simulink model "sampleModel226"  (R2021b)
settings: Solver=VariableStepAuto  StartTime=0.0  StopTime=10.0  RelTol=1e-3
undefined symbols (not defined in the file or in its folder): DiscIntNeverNeededParam, Newton, Raphson
libraries: simulink x16, slpidlib x3
settings Model: Creator=user  LastModifiedBy=user

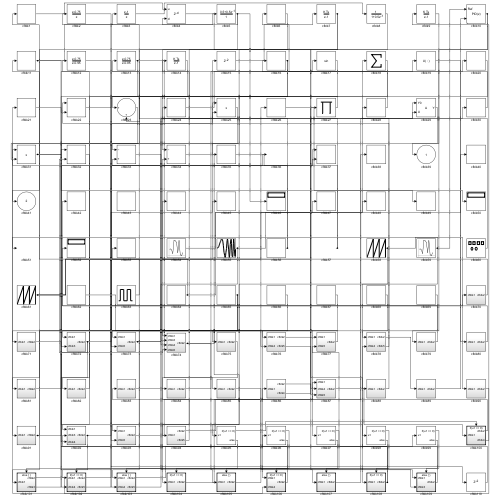
[thumbnail: Simulink's stored preview of the top-level diagram]
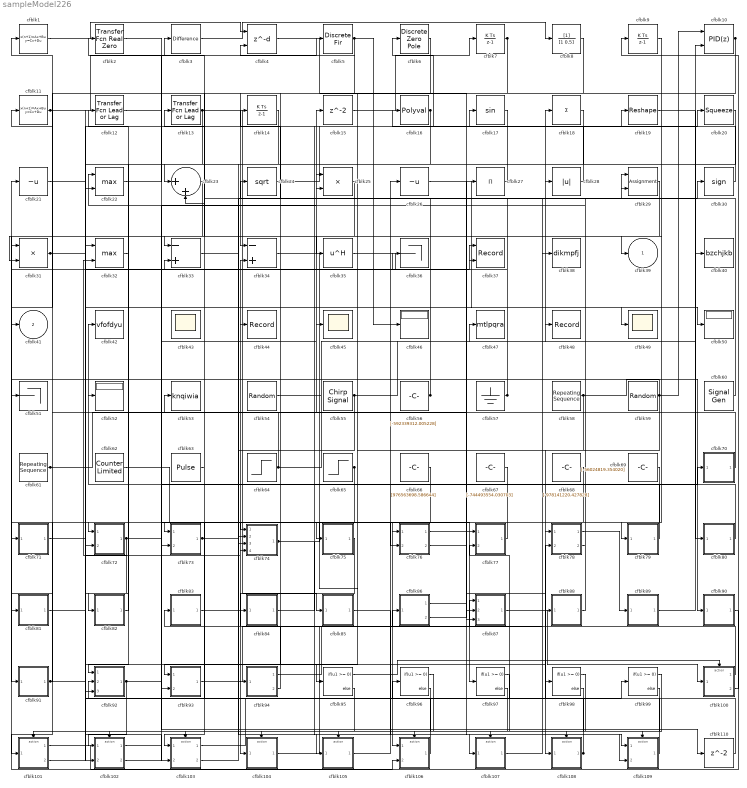
== system sampleModel226 ==
  cfblk1 : DiscreteStateSpace
  cfblk10 : slpidlib/PID Controller (2DOF)  Controller=PID  Form=Parallel  TimeDomain=Discrete-time  UseExternalTs=off  SampleTime=1  IntegratorMethod=Forward Euler  FilterMethod=Forward Euler  ControllerParametersSource=internal  P=1  I=1  D=0  UseFilter=on  N=100  b=1  c=1  TunerSelectOption=Transfer Function Based (PID Tuner App)  InitialConditionSource=internal  InitialConditionForIntegrator=0  InitialConditionForFilter=0  DifferentiatorICPrevScaledInput=0  ExternalReset=none  TrackingMode=off  Kt=1  LimitOutput=off  SatLimitsSource=internal  UpperSaturationLimit=inf  LowerSaturationLimit=-inf  LinearizeAsGain=off  AntiWindupMode=none  Kb=1  POutMin=[]  POutMax=[]  IOutMin=[]  IOutMax=[]  DOutMin=[]  DOutMax=[]  NOutMin=[]  NOutMax=[]  bOutMin=[]  bOutMax=[]  cOutMin=[]  cOutMax=[]  SumOutMin=[]  SumOutMax=[]  SaturationOutMin=[]  SaturationOutMax=[]  PParamMin=[]  PParamMax=[]  IParamMin=[]  IParamMax=[]  DParamMin=[]  DParamMax=[]  NParamMin=[]  NParamMax=[]  bParamMin=[]  bParamMax=[]  cParamMin=[]  cParamMax=[]  KbParamMin=[]  KbParamMax=[]  KtParamMin=[]  KtParamMax=[]  KbOutMin=[]  KbOutMax=[]  KtOutMin=[]  KtOutMax=[]  IntegratorOutMin=[]  IntegratorOutMax=[]  FilterOutMin=[]  FilterOutMax=[]  SumI1OutMin=[]  SumI1OutMax=[]  SumI2OutMin=[]  SumI2OutMax=[]  SumI3OutMin=[]  SumI3OutMax=[]  SumI4OutMin=[]  SumI4OutMax=[]  SumDOutMin=[]  SumDOutMax=[]  Sum1OutMin=[]  Sum1OutMax=[]  Sum2OutMin=[]  Sum2OutMax=[]  Sum3OutMin=[]  Sum3OutMax=[]  DifferentiatorOutMin=[]  DifferentiatorOutMax=[]  FilterDiffOutCoefMin=[]  FilterDiffOutCoefMax=[]  ReciprocalOutMin=[]  ReciprocalOutMax=[]  SumDenOutMin=[]  SumDenOutMax=[]  SumNumOutMin=[]  SumNumOutMax=[]  DivideOutMin=[]  DivideOutMax=[]  UdiffTsProdOutMin=[]  UdiffTsProdOutMax=[]  NTsProdOutMin=[]  NTsProdOutMax=[]  UintegralTsProdOutMin=[]  UintegralTsProdOutMax=[]  UngainTsProdOutMin=[]  UngainTsProdOutMax=[]  IntegratorContinuousStateAttributes=''  IntegratorStateMustResolveToSignalObject=off  IntegratorRTWStateStorageClass=Auto  FilterContinuousStateAttributes=''  FilterStateMustResolveToSignalObject=off  FilterRTWStateStorageClass=Auto  ParallelPVariant=InternalParameters  IdealPVariant=Disabled  IVariant=InternalParameters  DVariant=InternalParameters  bVariant=InternalParameters  cVariant=InternalParameters  IntegratorVariant=Discrete  SatVariant=Disabled  AWVariant=Passthrough  PCopyVariant=Disabled  TRVariant=Disabled  FdbkBlocksVariant=Forward  IdealPFdbkVariant=Disabled  SatFdbkVariant=Disabled  DerivativeFilterVariant=ForwardEulerFilter  NVariant=InternalParameters  NCopyVariant=Disabled  FilterICVariant=InternalICsFilter  IntegratorICVariant=InternalICs  ExternalResetVariant=Disabled  TRSumVariant=Passthrough  SumFdbkVariant=Disabled  SumVariant=Sum_PID  TsampFilterVariant=InternalTs  TsampNgainVariant=Passthrough  TsampIntegralVariant=Passthrough  ExternalSaturationOutDataTypeStr=Inherit: Same as second input
      settings: SourceProductBaseCode=SL
  cfblk100 : Subsystem  TreatAsAtomicUnit=on
  cfblk101 : Subsystem  TreatAsAtomicUnit=on
  cfblk102 : Subsystem  TreatAsAtomicUnit=on
  cfblk103 : Subsystem  TreatAsAtomicUnit=on
  cfblk104 : Subsystem  TreatAsAtomicUnit=on
  cfblk105 : Subsystem  TreatAsAtomicUnit=on
  cfblk106 : Subsystem  TreatAsAtomicUnit=on
  cfblk107 : Subsystem  TreatAsAtomicUnit=on
  cfblk108 : Subsystem  TreatAsAtomicUnit=on
  cfblk109 : Subsystem  TreatAsAtomicUnit=on
  cfblk11 : DiscreteStateSpace
  cfblk110 : Delay  SampleTime=1
  cfblk12 : simulink/Discrete/Transfer Fcn Lead or Lag  PoleZ=0.95  ZeroZ=0.75  ICPrevOutput=0.0  ICPrevInput=0.0  DoSatur=off
      settings: SourceProductBaseCode=SL
  cfblk13 : simulink/Discrete/Transfer Fcn Lead or Lag  PoleZ=0.95  ZeroZ=0.75  ICPrevOutput=0.0  ICPrevInput=0.0  DoSatur=off
      settings: SourceProductBaseCode=SL
  cfblk14 : DiscreteIntegrator  ICPrevOutput=DiscIntNeverNeededParam  ICPrevScaledInput=DiscIntNeverNeededParam
  cfblk15 : Delay  SampleTime=1
  cfblk16 : Polyval  Coefs=[ +2.081618890e-019, -1.441693666e-014, +4.719686976e-010, -8.536869453e-006, +1.621573104e-001, -8.087801117e+001 ]
  cfblk17 : Trigonometry
  cfblk18 : Sum  Inputs=+
  cfblk19 : Reshape
  cfblk2 : simulink/Discrete/Transfer Fcn Real Zero  ZeroZ=0.75  ICPrevInput=0.0  DoSatur=off
      settings: SourceProductBaseCode=SL
  cfblk20 : Squeeze
  cfblk21 : UnaryMinus
  cfblk22 : MinMax  Function=max  Inputs=2
  cfblk23 : Sum  Inputs=|++
  cfblk24 : Sqrt  SaturateOnIntegerOverflow=on
  cfblk25 : Product
  cfblk26 : UnaryMinus
  cfblk27 : Product  Inputs=*
  cfblk28 : Abs
  cfblk29 : Assignment  DiagnosticForDimensions=Warning  IndexOptions=Index vector (dialog)  Indices=1  OutputSizes=1
  cfblk3 : simulink/Discrete/Difference  ICPrevInput=0.0  OutMin=[]  OutMax=[]  OutDataTypeStr=Inherit: Inherit via back propagation  OutDataType=fixdt(1, 16)  OutScaling=2^-10  DoSatur=off
  cfblk30 : Signum
  cfblk31 : Product  Inputs=**
  cfblk32 : MinMax  Function=max  Inputs=2
  cfblk33 : Sum  Inputs=-+
  cfblk34 : Sum  Inputs=-+
  cfblk35 : Math  Operator=hermitian  SaturateOnIntegerOverflow=on
  cfblk36 : Terminator
  cfblk37 : Record  FileSettingsInternal="{\"entries\":[{\"content\":{\"excelSettings\":{\"content\":{},\"type\":\"Streamout.ExcelSettings\"}},\"type\":\"Streamout.FileSettingStorage\",\"uuid\":\"d36e2a6a-7d58-4cca-bbfa-2d4460a6e9a2\"}],\"packageUris\":[\"http://schema.mathworks.com/mf0/streamout_blocks/R2020a\"],\"version\":\"1.0\"}"  Layout=[1 1]  SignalsInternal="{\"entries\":[{\"content\":{\"signals\":[{\"content\":{\"blockPath\":[\"sampleModel226/cfblk37\"],\"channel\":[],\"dimensions\":[1],\"domain\":\"sampleModel226/cfblk37\",\"lineColor\":\"#a2142f\",\"plots\":[1],\"port\":1,\"sid\":[\"\"],\"signalID\":8845,\"signalName\":\"cfblk81\"},\"type\":\"RecordBlkView.Signal\",\"uuid\":\"4bfdb0e3-98e3-43bb-8b1d-080535746a11\"},{\"content\":{\"blockPath\":[\"sampleModel226/cfblk37\"],\"channel\":[],\"dimensions\":[1,1],\"domain\":\"sampleModel226/cfblk37\",\"lineColor\":\"#139fff\",\"plots\":[1],\"port\":2,\"sid\":[\"\"],\"signalID\":8849,\"signalName\":\"cfblk35\"},\"type\":\"RecordBlkView.Signal\",\"uuid\":\"6c2a1cae-b381-4225-acec-e32f350de892\"}]},\"type\":\"RecordBlkView.InputSignals\",\"uuid\":\"7360f588-8737-44e8-b6c5-5c4f20366708\"}],\"packageUris\":[\"http://schema.mathworks.com/mf0/streamout_blocks/R2020a\"],\"version\":\"1.0\"}"  VisualizationBindings="{\"xyplotplugin\":{\"info\":[{\"series\":[{\"bindingParametersList\":[{\"parameter\":\"X-Axis\",\"signalID\":8845,\"signalName\":\"cfblk81\"},{\"parameter\":\"Y-Axis\",\"signalID\":8849,\"signalName\":\"cfblk35\"}],\"seriesID\":61832}],\"subplotID\":1}]}}"  CompatibilityTag=XY
  cfblk38 : ToWorkspace  VariableName=dikmpfj  SaveFormat=Timeseries  SampleTime=-1
  cfblk4 : Delay  DelayLengthSource=Input port  SampleTime=1
      settings: InputPortMap=u0,p1
  cfblk40 : ToWorkspace  VariableName=bzchjkb  SaveFormat=Timeseries  SampleTime=-1
  cfblk42 : ToWorkspace  VariableName=vfofdyu  SaveFormat=Timeseries  SampleTime=-1
  cfblk43 : Scope
      settings: Floating=on
  cfblk44 : Record  FileSettingsInternal="{\"entries\":[{\"content\":{\"excelSettings\":{\"content\":{},\"type\":\"Streamout.ExcelSettings\"}},\"type\":\"Streamout.FileSettingStorage\",\"uuid\":\"6da709ca-63db-447c-bae5-9ad803eba82c\"}],\"packageUris\":[\"http://schema.mathworks.com/mf0/streamout_blocks/R2020a\"],\"version\":\"1.0\"}"  SignalsInternal="{\"entries\":[{\"content\":{\"signals\":[{\"content\":{\"blockPath\":[\"sampleModel226/cfblk44\"],\"channel\":[],\"dimensions\":[1],\"domain\":\"sampleModel226/cfblk44\",\"lineColor\":\"#64d413\",\"plots\":[1],\"port\":1,\"sid\":[\"\"],\"signalID\":8853,\"signalName\":\"cfblk70\"},\"type\":\"RecordBlkView.Signal\",\"uuid\":\"6e64be09-163b-49ba-8a46-496ddf1f160c\"}]},\"type\":\"RecordBlkView.InputSignals\",\"uuid\":\"22720668-7b37-4b9a-8f54-b019708bc10f\"}],\"packageUris\":[\"http://schema.mathworks.com/mf0/streamout_blocks/R2020a\"],\"version\":\"1.0\"}"  VisualizationBindings="{\"sparklinesplugin\":{\"info\":[{\"bindingParametersList\":[],\"subplotID\":1}]}}"
  cfblk45 : Scope
  cfblk46 : Display
  cfblk47 : ToWorkspace  VariableName=mtlpqra  SaveFormat=Timeseries  SampleTime=-1
  cfblk48 : Record  FileSettingsInternal="{\"entries\":[{\"content\":{\"excelSettings\":{\"content\":{},\"type\":\"Streamout.ExcelSettings\"}},\"type\":\"Streamout.FileSettingStorage\",\"uuid\":\"889c16d3-eb07-45b4-991a-61aa03e04959\"}],\"packageUris\":[\"http://schema.mathworks.com/mf0/streamout_blocks/R2020a\"],\"version\":\"1.0\"}"  SignalsInternal="{\"entries\":[{\"content\":{\"signals\":[{\"content\":{\"blockPath\":[\"sampleModel226/cfblk48\"],\"channel\":[],\"dimensions\":[1],\"domain\":\"sampleModel226/cfblk48\",\"lineColor\":\"#ff13a6\",\"plots\":[1],\"port\":1,\"sid\":[\"\"],\"signalID\":8857,\"signalName\":\"cfblk105\"},\"type\":\"RecordBlkView.Signal\",\"uuid\":\"d455fa8b-51d8-45b8-9a0a-93b8cc8b601d\"}]},\"type\":\"RecordBlkView.InputSignals\",\"uuid\":\"c71b9389-408f-46ae-9f87-9ca061c3a80b\"}],\"packageUris\":[\"http://schema.mathworks.com/mf0/streamout_blocks/R2020a\"],\"version\":\"1.0\"}"  VisualizationBindings="{\"sparklinesplugin\":{\"info\":[{\"bindingParametersList\":[],\"subplotID\":1}]}}"
  cfblk49 : Scope
  cfblk5 : DiscreteFir  SampleTime=1
  cfblk50 : Display
  cfblk51 : Terminator
  cfblk52 : Display
  cfblk53 : ToWorkspace  VariableName=knqiwia  SaveFormat=Timeseries  SampleTime=-1
  cfblk54 : RandomNumber  Mean=[-4325.746459]  Variance=[71427.847136]  Seed=[10241733.000000]  SampleTime=0.1
  cfblk55 : simulink/Sources/Chirp Signal  f1=[915626819.225968]  T=[-611916928.830304]  f2=[289527233.085655]
  cfblk56 : Constant  Value=[-592339312.005228]  SampleTime=1
  cfblk57 : Ground
  cfblk58 : simulink/Sources/Repeating Sequence  rep_seq_t=[0 2]  rep_seq_y=[-226440358.666034, 924879939.640409]
  cfblk59 : RandomNumber  Mean=[-93942.652973]  Variance=[96041.707284]  Seed=[790619.000000]  SampleTime=0.1
  cfblk6 : DiscreteZeroPole  Poles=[0 0.5]  Gain=1
  cfblk60 : SignalGenerator  Amplitude=[693207855.217041]  Units=rad/sec
  cfblk61 : simulink/Sources/Repeating Sequence  rep_seq_t=[0 2]  rep_seq_y=[41982134.233435, 527034416.081675]
  cfblk62 : simulink/Sources/Counter Limited  uplimit=[765.000000]  tsamp=-1
  cfblk63 : DiscretePulseGenerator  PulseType=Time based  Amplitude=[-918031499.996317]  Period=[48545849.790406]  PulseWidth=5  PhaseDelay=[2.000000]
  cfblk64 : Step  Time=[49.000000]  Before=[-570561474.659156]  After=[998963794.152262]  SampleTime=0
  cfblk65 : Step  Time=[40.000000]  Before=[357232661.862579]  After=[745987959.330450]  SampleTime=0
  cfblk66 : Constant  Value=[976563698.586644]  SampleTime=1
  cfblk67 : Constant  Value=[-744493554.030703]  SampleTime=1
  cfblk68 : Constant  Value=[-978141220.427828]  SampleTime=1
  cfblk69 : Constant  Value=[-56024819.354020]  SampleTime=1
  cfblk7 : DiscreteIntegrator  ICPrevOutput=DiscIntNeverNeededParam  ICPrevScaledInput=DiscIntNeverNeededParam
  cfblk70 : Subsystem
  cfblk71 : Subsystem
  cfblk72 : Subsystem
  cfblk73 : Subsystem
  cfblk74 : Subsystem
  cfblk75 : Subsystem
  cfblk76 : Subsystem
  cfblk77 : Subsystem
  cfblk78 : Subsystem
  cfblk79 : Subsystem
  cfblk8 : DiscreteFilter  SampleTime=1
  cfblk80 : Subsystem
  cfblk81 : Subsystem
  cfblk82 : Subsystem
  cfblk83 : Subsystem
  cfblk84 : Subsystem
  cfblk85 : Subsystem
  cfblk86 : Subsystem
  cfblk87 : Subsystem
  cfblk88 : Subsystem
  cfblk89 : Subsystem
  cfblk9 : DiscreteIntegrator  ICPrevOutput=DiscIntNeverNeededParam  ICPrevScaledInput=DiscIntNeverNeededParam
  cfblk90 : Subsystem
  cfblk91 : Subsystem
  cfblk92 : Subsystem
  cfblk93 : Subsystem
  cfblk94 : Subsystem
  cfblk{95..99} (5 alike) : If  IfExpression=u1 >= 0  SampleTime=1
  cfblk39 : Outport
  cfblk41 : Outport  Port=2
  wires:
  cfblk11/1 -> cfblk3/1, cfblk50/1
  cfblk13/1 -> cfblk85/1(cfblk1), cfblk22/2
  cfblk24/1 -> cfblk19/1
  cfblk27/1 -> cfblk23/1
  cfblk3/1 -> cfblk8/1
  cfblk87/1(cfblk2) -> cfblk100/1(cfblk1)
  cfblk26/1 -> cfblk49/1
  cfblk59/1 -> cfblk108/1(cfblk1), cfblk51/1, cfblk10/1
  cfblk34/1 -> cfblk93/1(cfblk1)
  cfblk90/1(cfblk2) -> cfblk21/1
  cfblk58/1 -> cfblk90/1(cfblk1), cfblk95/1
  cfblk69/1 -> cfblk106/1(cfblk1)
  cfblk15/1 -> cfblk7/1
  cfblk23/1 -> cfblk91/1(cfblk1)
  cfblk77/1(cfblk2) -> cfblk72/1(cfblk1)
  cfblk68/1 -> cfblk78/1(cfblk1)
  cfblk72/1(cfblk2) -> cfblk32/2, cfblk92/3(cfblk4), cfblk36/1
  cfblk74/1(cfblk2) -> cfblk76/1(cfblk1), cfblk109/2(cfblk3)
  cfblk7/1 -> cfblk34/1, cfblk33/1
  cfblk104/1(cfblk2) -> cfblk86/1(cfblk1)
  cfblk64/1 -> cfblk47/1, cfblk11/1
  cfblk1/1 -> cfblk4/1
  cfblk65/1 -> cfblk71/1(cfblk1), cfblk81/1(cfblk1), cfblk73/1(cfblk1)
  cfblk14/1 -> cfblk23/2
  cfblk62/1 -> cfblk97/1
  cfblk101/1(cfblk2) -> cfblk106/2(cfblk4)
  cfblk83/1(cfblk2) -> cfblk34/2
  cfblk103/1(cfblk2) -> cfblk99/1
  cfblk109/1(cfblk2) -> cfblk78/2(cfblk4)
  cfblk31/1 -> cfblk20/1, cfblk103/2(cfblk4)
  cfblk61/1 -> cfblk15/1, cfblk27/1, cfblk26/1
  cfblk6/1 -> cfblk41/1
  cfblk56/1 -> cfblk31/1, cfblk14/1
  cfblk92/1(cfblk2) -> cfblk102/1(cfblk1), cfblk25/2
  cfblk107/1(cfblk2) -> cfblk29/1
  cfblk75/1(cfblk2) -> cfblk104/1(cfblk1)
  cfblk19/1 -> cfblk80/1(cfblk1)
  cfblk80/1(cfblk2) -> cfblk42/1
  cfblk91/1(cfblk2) -> cfblk1/1, cfblk74/4(cfblk5)
  cfblk2/1 -> cfblk74/1(cfblk1)
  cfblk70/1(cfblk2) -> cfblk44/1
  cfblk55/1 -> cfblk74/2(cfblk3), cfblk10/2
  cfblk54/1 -> cfblk18/1
  cfblk4/1 -> cfblk77/1(cfblk1)
  cfblk93/1(cfblk2) -> cfblk87/1(cfblk1)
  cfblk28/1 -> cfblk16/1
  cfblk10/1 -> cfblk79/1(cfblk1), cfblk87/3(cfblk5)
  cfblk106/1(cfblk2) -> cfblk83/1(cfblk1)
  cfblk88/1(cfblk2) -> cfblk28/1
  cfblk78/1(cfblk2) -> cfblk89/1(cfblk1)
  cfblk108/1(cfblk2) -> cfblk77/2(cfblk5), cfblk92/2(cfblk3)
  cfblk21/1 -> cfblk72/2(cfblk3)
  cfblk94/1(cfblk2) -> cfblk38/1
  cfblk105/1(cfblk2) -> cfblk48/1
  cfblk67/1 -> cfblk103/1(cfblk1)
  cfblk32/1 -> cfblk82/1(cfblk1)
  cfblk57/1 -> cfblk2/1, cfblk33/2
  cfblk82/1(cfblk2) -> cfblk12/1
  cfblk25/1 -> cfblk102/2(cfblk4)
  cfblk29/1 -> cfblk31/2
  cfblk71/1(cfblk2) -> cfblk98/1
  cfblk17/1 -> cfblk92/1(cfblk1)
  cfblk22/1 -> cfblk5/1
  cfblk33/1 -> cfblk76/2(cfblk4)
  cfblk101/2(cfblk3) -> cfblk96/1
  cfblk76/1(cfblk2) -> cfblk109/1(cfblk1)
  cfblk94/2(cfblk5) -> cfblk84/1(cfblk1)
  cfblk60/1 -> cfblk24/1
  cfblk63/1 -> cfblk13/1
  cfblk8/1 -> cfblk75/1(cfblk1)
  cfblk5/1 -> cfblk94/1(cfblk1), cfblk4/2, cfblk46/1
  cfblk103/2(cfblk5) -> cfblk25/1
  cfblk18/1 -> cfblk74/3(cfblk4)
  cfblk81/1(cfblk2) -> cfblk37/1
  cfblk20/1 -> cfblk35/1
  cfblk66/1 -> cfblk101/1(cfblk1)
  cfblk73/1(cfblk2) -> cfblk105/1(cfblk1), cfblk29/2
  cfblk100/1(cfblk2) -> cfblk53/1
  cfblk16/1 -> cfblk93/2(cfblk5), cfblk73/2(cfblk5)
  cfblk9/1 -> cfblk39/1
  cfblk89/1(cfblk2) -> cfblk40/1
  cfblk76/2(cfblk5) -> cfblk88/1(cfblk1)
  cfblk86/1(cfblk2) -> cfblk87/2(cfblk4)
  cfblk78/2(cfblk5) -> cfblk22/1
  cfblk85/1(cfblk2) -> cfblk107/1(cfblk1)
  cfblk35/1 -> cfblk37/2
  cfblk30/1 -> cfblk6/1
  cfblk86/2(cfblk4) -> cfblk30/1
  cfblk84/1(cfblk2) -> cfblk17/1
  cfblk100/2(cfblk4) -> cfblk9/1
  cfblk102/1(cfblk2) -> cfblk45/1
  cfblk102/2(cfblk5) -> cfblk70/1(cfblk1)
  cfblk79/1(cfblk2) -> cfblk52/1
  cfblk95/1 -> cfblk100/Action
  cfblk95/2 -> cfblk101/Action
  cfblk96/1 -> cfblk102/Action
  cfblk96/2 -> cfblk103/Action
  cfblk97/1 -> cfblk104/Action
  cfblk97/2 -> cfblk105/Action
  cfblk98/1 -> cfblk106/Action
  cfblk98/2 -> cfblk107/Action
  cfblk99/1 -> cfblk108/Action
  cfblk99/2 -> cfblk109/Action
  cfblk12/1 -> cfblk110/1
  cfblk110/1 -> cfblk32/1

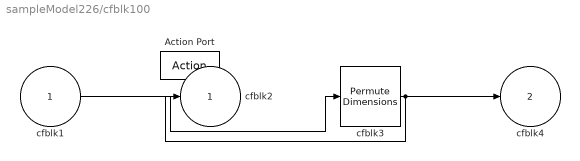
== system sampleModel226/cfblk100 ==
  cfblk1 : Inport
  Action Port : ActionPort  ActionPortLabel=if(u1 >= 0)
  cfblk3 : PermuteDimensions
  cfblk2 : Outport
  cfblk4 : Outport  Port=2
  wires:
  cfblk1/1 -> cfblk3/1
  cfblk3/1 -> cfblk2/1, cfblk4/1

== system sampleModel226/cfblk101 ==
  cfblk1 : Inport
  Action Port : ActionPort  ActionPortLabel=else
  cfblk2 : Outport
  cfblk3 : Outport  Port=2
  wires:
  cfblk1/1 -> cfblk2/1, cfblk3/1

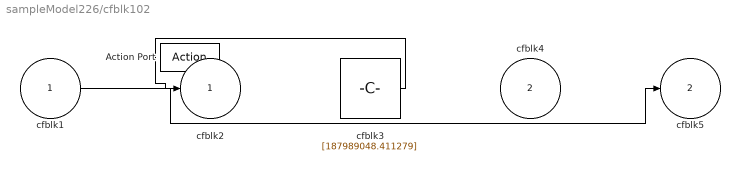
== system sampleModel226/cfblk102 ==
  cfblk1 : Inport
  cfblk4 : Inport  Port=2
  Action Port : ActionPort  ActionPortLabel=if(u1 >= 0)
  cfblk3 : Constant  Value=[187989048.411279]  SampleTime=1
  cfblk2 : Outport
  cfblk5 : Outport  Port=2
  wires:
  cfblk1/1 -> cfblk5/1
  cfblk3/1 -> cfblk2/1

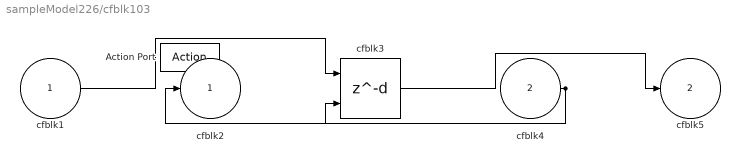
== system sampleModel226/cfblk103 ==
  cfblk1 : Inport
  cfblk4 : Inport  Port=2
  Action Port : ActionPort  ActionPortLabel=else
  cfblk3 : Delay  DelayLengthSource=Input port
      settings: InputPortMap=u0,p1
  cfblk2 : Outport
  cfblk5 : Outport  Port=2
  wires:
  cfblk3/1 -> cfblk5/1
  cfblk4/1 -> cfblk2/1, cfblk3/2
  cfblk1/1 -> cfblk3/1

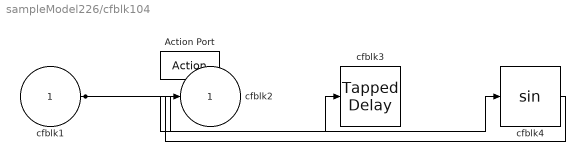
== system sampleModel226/cfblk104 ==
  cfblk1 : Inport
  Action Port : ActionPort  ActionPortLabel=if(u1 >= 0)
  cfblk3 : simulink/Discrete/Tapped Delay  vinit=0.0  samptime=-1  NumDelays=1  DelayOrder=Oldest  includeCurrent=off
  cfblk4 : Trigonometry
  cfblk2 : Outport
  wires:
  cfblk1/1 -> cfblk4/1, cfblk3/1
  cfblk4/1 -> cfblk2/1

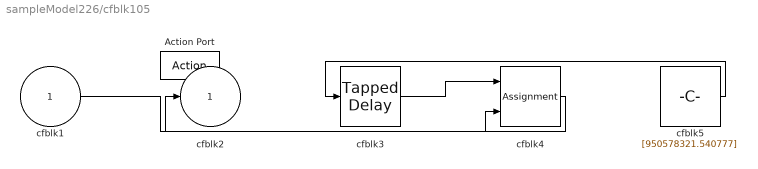
== system sampleModel226/cfblk105 ==
  cfblk1 : Inport
  Action Port : ActionPort  ActionPortLabel=else
  cfblk3 : simulink/Discrete/Tapped Delay  vinit=0.0  samptime=-1  NumDelays=1  DelayOrder=Oldest  includeCurrent=off
  cfblk4 : Assignment  DiagnosticForDimensions=Warning  IndexOptions=Index vector (dialog)  Indices=1  OutputSizes=1
  cfblk5 : Constant  Value=[950578321.540777]  SampleTime=1
  cfblk2 : Outport
  wires:
  cfblk4/1 -> cfblk2/1
  cfblk5/1 -> cfblk3/1
  cfblk3/1 -> cfblk4/1
  cfblk1/1 -> cfblk4/2

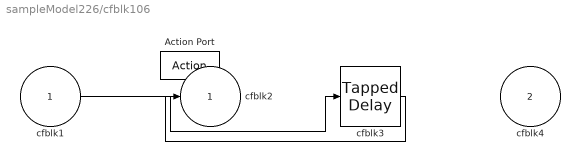
== system sampleModel226/cfblk106 ==
  cfblk1 : Inport
  cfblk4 : Inport  Port=2
  Action Port : ActionPort  ActionPortLabel=if(u1 >= 0)
  cfblk3 : simulink/Discrete/Tapped Delay  vinit=0.0  samptime=-1  NumDelays=1  DelayOrder=Oldest  includeCurrent=off
  cfblk2 : Outport
  wires:
  cfblk1/1 -> cfblk3/1
  cfblk3/1 -> cfblk2/1

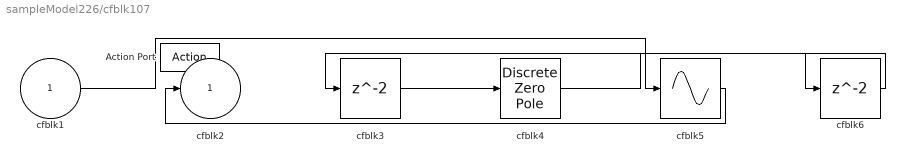
== system sampleModel226/cfblk107 ==
  cfblk1 : Inport
  Action Port : ActionPort  ActionPortLabel=else
  cfblk3 : Delay
  cfblk4 : DiscreteZeroPole  Poles=[0 0.5]  Gain=1  SampleTime=-1
  cfblk5 : Sin  TimeSource=Use external signal  SampleTime=0
  cfblk6 : Delay
  cfblk2 : Outport
  wires:
  cfblk5/1 -> cfblk2/1
  cfblk1/1 -> cfblk5/1
  cfblk3/1 -> cfblk4/1
  cfblk4/1 -> cfblk6/1
  cfblk6/1 -> cfblk3/1

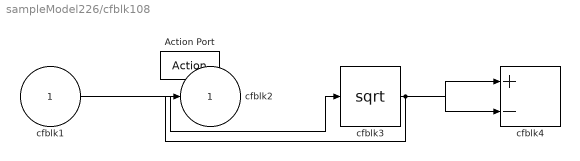
== system sampleModel226/cfblk108 ==
  cfblk1 : Inport
  Action Port : ActionPort  ActionPortLabel=if(u1 >= 0)
  cfblk3 : Sqrt  SaturateOnIntegerOverflow=on
  cfblk4 : Sum  Inputs=+-
  cfblk2 : Outport
  wires:
  cfblk1/1 -> cfblk3/1
  cfblk3/1 -> cfblk2/1, cfblk4/1, cfblk4/2

== system sampleModel226/cfblk109 ==
  cfblk1 : Inport
  cfblk3 : Inport  Port=2
  Action Port : ActionPort  ActionPortLabel=else
  cfblk2 : Outport
  wires:
  cfblk3/1 -> cfblk2/1

== system sampleModel226/cfblk70 ==
  cfblk1 : Inport
  cfblk3 : Product  Inputs=*
  cfblk2 : Outport
  wires:
  cfblk1/1 -> cfblk3/1
  cfblk3/1 -> cfblk2/1

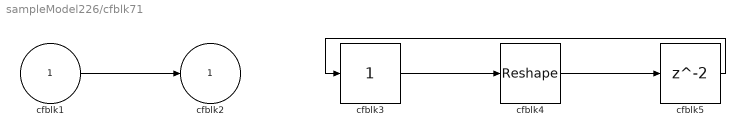
== system sampleModel226/cfblk71 ==
  cfblk1 : Inport
  cfblk3 : simulink/Math Operations/Slider Gain  gain=1  low=0  high=2
  cfblk4 : Reshape
  cfblk5 : Delay  SampleTime=1
  cfblk2 : Outport
  wires:
  cfblk1/1 -> cfblk2/1
  cfblk3/1 -> cfblk4/1
  cfblk4/1 -> cfblk5/1
  cfblk5/1 -> cfblk3/1

== system sampleModel226/cfblk72 ==
  cfblk1 : Inport
  cfblk3 : Inport  Port=2
  cfblk2 : Outport
  wires:
  cfblk3/1 -> cfblk2/1

== system sampleModel226/cfblk73 ==
  cfblk1 : Inport
  cfblk5 : Inport  Port=2
  cfblk3 : slpidlib/PID Controller (2DOF)  Controller=PID  Form=Parallel  TimeDomain=Discrete-time  UseExternalTs=off  SampleTime=1  IntegratorMethod=Forward Euler  FilterMethod=Forward Euler  ControllerParametersSource=internal  P=1  I=1  D=0  UseFilter=on  N=100  b=1  c=1  TunerSelectOption=Transfer Function Based (PID Tuner App)  InitialConditionSource=internal  InitialConditionForIntegrator=0  InitialConditionForFilter=0  DifferentiatorICPrevScaledInput=0  ExternalReset=none  TrackingMode=off  Kt=1  LimitOutput=off  SatLimitsSource=internal  UpperSaturationLimit=inf  LowerSaturationLimit=-inf  LinearizeAsGain=off  AntiWindupMode=none  Kb=1  POutMin=[]  POutMax=[]  IOutMin=[]  IOutMax=[]  DOutMin=[]  DOutMax=[]  NOutMin=[]  NOutMax=[]  bOutMin=[]  bOutMax=[]  cOutMin=[]  cOutMax=[]  SumOutMin=[]  SumOutMax=[]  SaturationOutMin=[]  SaturationOutMax=[]  PParamMin=[]  PParamMax=[]  IParamMin=[]  IParamMax=[]  DParamMin=[]  DParamMax=[]  NParamMin=[]  NParamMax=[]  bParamMin=[]  bParamMax=[]  cParamMin=[]  cParamMax=[]  KbParamMin=[]  KbParamMax=[]  KtParamMin=[]  KtParamMax=[]  KbOutMin=[]  KbOutMax=[]  KtOutMin=[]  KtOutMax=[]  IntegratorOutMin=[]  IntegratorOutMax=[]  FilterOutMin=[]  FilterOutMax=[]  SumI1OutMin=[]  SumI1OutMax=[]  SumI2OutMin=[]  SumI2OutMax=[]  SumI3OutMin=[]  SumI3OutMax=[]  SumI4OutMin=[]  SumI4OutMax=[]  SumDOutMin=[]  SumDOutMax=[]  Sum1OutMin=[]  Sum1OutMax=[]  Sum2OutMin=[]  Sum2OutMax=[]  Sum3OutMin=[]  Sum3OutMax=[]  DifferentiatorOutMin=[]  DifferentiatorOutMax=[]  FilterDiffOutCoefMin=[]  FilterDiffOutCoefMax=[]  ReciprocalOutMin=[]  ReciprocalOutMax=[]  SumDenOutMin=[]  SumDenOutMax=[]  SumNumOutMin=[]  SumNumOutMax=[]  DivideOutMin=[]  DivideOutMax=[]  UdiffTsProdOutMin=[]  UdiffTsProdOutMax=[]  NTsProdOutMin=[]  NTsProdOutMax=[]  UintegralTsProdOutMin=[]  UintegralTsProdOutMax=[]  UngainTsProdOutMin=[]  UngainTsProdOutMax=[]  IntegratorContinuousStateAttributes=''  IntegratorStateMustResolveToSignalObject=off  IntegratorRTWStateStorageClass=Auto  FilterContinuousStateAttributes=''  FilterStateMustResolveToSignalObject=off  FilterRTWStateStorageClass=Auto  ParallelPVariant=InternalParameters  IdealPVariant=Disabled  IVariant=InternalParameters  DVariant=InternalParameters  bVariant=InternalParameters  cVariant=InternalParameters  IntegratorVariant=Discrete  SatVariant=Disabled  AWVariant=Passthrough  PCopyVariant=Disabled  TRVariant=Disabled  FdbkBlocksVariant=Forward  IdealPFdbkVariant=Disabled  SatFdbkVariant=Disabled  DerivativeFilterVariant=ForwardEulerFilter  NVariant=InternalParameters  NCopyVariant=Disabled  FilterICVariant=InternalICsFilter  IntegratorICVariant=InternalICs  ExternalResetVariant=Disabled  TRSumVariant=Passthrough  SumFdbkVariant=Disabled  SumVariant=Sum_PID  TsampFilterVariant=InternalTs  TsampNgainVariant=Passthrough  TsampIntegralVariant=Passthrough  ExternalSaturationOutDataTypeStr=Inherit: Same as second input
      settings: SourceProductBaseCode=SL
  cfblk4 : Polyval  Coefs=[ +2.081618890e-019, -1.441693666e-014, +4.719686976e-010, -8.536869453e-006, +1.621573104e-001, -8.087801117e+001 ]
  cfblk2 : Outport
  wires:
  cfblk4/1 -> cfblk2/1
  cfblk1/1 -> cfblk4/1
  cfblk5/1 -> cfblk3/1, cfblk3/2

== system sampleModel226/cfblk74 ==
  cfblk1 : Inport
  cfblk3 : Inport  Port=2
  cfblk4 : Inport  Port=3
  cfblk5 : Inport  Port=4
  cfblk2 : Outport
  wires:
  cfblk1/1 -> cfblk2/1

== system sampleModel226/cfblk75 ==
  cfblk1 : Inport
  cfblk3 : Sum  Inputs=|++
  cfblk4 : Abs
  cfblk5 : Delay  SampleTime=1
  cfblk2 : Outport
  wires:
  cfblk1/1 -> cfblk3/1
  cfblk4/1 -> cfblk2/1, cfblk5/1
  cfblk3/1 -> cfblk4/1
  cfblk5/1 -> cfblk3/2

== system sampleModel226/cfblk76 ==
  cfblk1 : Inport
  cfblk4 : Inport  Port=2
  cfblk3 : Product  Inputs=**
  cfblk2 : Outport
  cfblk5 : Outport  Port=2
  wires:
  cfblk1/1 -> cfblk3/1
  cfblk3/1 -> cfblk5/1
  cfblk4/1 -> cfblk2/1, cfblk3/2

== system sampleModel226/cfblk77 ==
  cfblk1 : Inport
  cfblk5 : Inport  Port=2
  cfblk3 : simulink/Discrete/Difference  ICPrevInput=0.0  OutMin=[]  OutMax=[]  OutDataTypeStr=Inherit: Inherit via back propagation  OutDataType=fixdt(1, 16)  OutScaling=2^-10  DoSatur=off
  cfblk4 : Constant  Value=[-267108798.148476]  SampleTime=1
  cfblk2 : Outport
  wires:
  cfblk5/1 -> cfblk3/1
  cfblk4/1 -> cfblk2/1

== system sampleModel226/cfblk78 ==
  cfblk1 : Inport
  cfblk4 : Inport  Port=2
  cfblk3 : Reshape
  cfblk2 : Outport
  cfblk5 : Outport  Port=2
  wires:
  cfblk1/1 -> cfblk5/1
  cfblk4/1 -> cfblk3/1
  cfblk3/1 -> cfblk2/1

== system sampleModel226/cfblk79 ==
  cfblk1 : Inport
  cfblk3 : Sum  Inputs=|++
  cfblk4 : Sqrt  Operator=rSqrt  AlgorithmType=Newton-Raphson  SaturateOnIntegerOverflow=on
  cfblk5 : Constant  Value=[428157044.886283]  SampleTime=1
  cfblk2 : Outport
  wires:
  cfblk4/1 -> cfblk2/1
  cfblk3/1 -> cfblk4/1
  cfblk1/1 -> cfblk3/1
  cfblk5/1 -> cfblk3/2

== system sampleModel226/cfblk80 ==
  cfblk1 : Inport
  cfblk3 : simulink/Math Operations/MinMax Running Resettable  Function=min  vinit=0.0
  cfblk2 : Outport
  wires:
  cfblk1/1 -> cfblk3/1, cfblk3/2
  cfblk3/1 -> cfblk2/1

== system sampleModel226/cfblk81 ==
  cfblk1 : Inport
  cfblk3 : ComplexToMagnitudeAngle
  cfblk2 : Outport
  wires:
  cfblk3/1 -> cfblk2/1
  cfblk1/1 -> cfblk3/1

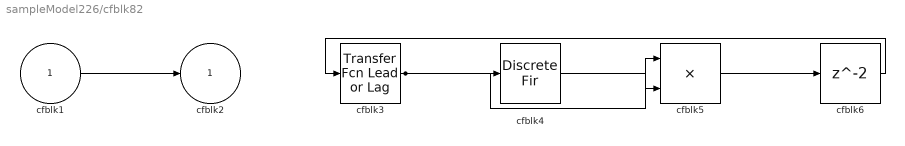
== system sampleModel226/cfblk82 ==
  cfblk1 : Inport
  cfblk3 : simulink/Discrete/Transfer Fcn Lead or Lag  PoleZ=0.95  ZeroZ=0.75  ICPrevOutput=0.0  ICPrevInput=0.0  DoSatur=off
      settings: SourceProductBaseCode=SL
  cfblk4 : DiscreteFir  SampleTime=1
  cfblk5 : Product
  cfblk6 : Delay  SampleTime=1
  cfblk2 : Outport
  wires:
  cfblk1/1 -> cfblk2/1
  cfblk3/1 -> cfblk5/1, cfblk4/1
  cfblk4/1 -> cfblk5/2
  cfblk5/1 -> cfblk6/1
  cfblk6/1 -> cfblk3/1

== system sampleModel226/cfblk83 ==
  cfblk1 : Inport
  cfblk3 : DiscreteIntegrator  ICPrevOutput=DiscIntNeverNeededParam  ICPrevScaledInput=DiscIntNeverNeededParam
  cfblk4 : Bias  Bias=[908485912.588016]
  cfblk2 : Outport
  wires:
  cfblk4/1 -> cfblk2/1
  cfblk3/1 -> cfblk4/1
  cfblk1/1 -> cfblk3/1

== system sampleModel226/cfblk84 ==
  cfblk1 : Inport
  cfblk3 : Product  Inputs=**
  cfblk4 : Constant  Value=[-65304025.086890]  SampleTime=1
  cfblk2 : Outport
  wires:
  cfblk3/1 -> cfblk2/1
  cfblk1/1 -> cfblk3/1
  cfblk4/1 -> cfblk3/2

== system sampleModel226/cfblk85 ==
  cfblk1 : Inport
  cfblk3 : DiscreteTransferFcn  SampleTime=1
  cfblk2 : Outport
  wires:
  cfblk1/1 -> cfblk2/1, cfblk3/1

== system sampleModel226/cfblk86 ==
  cfblk1 : Inport
  cfblk3 : Sum  Inputs=+-
  cfblk2 : Outport
  cfblk4 : Outport  Port=2
  wires:
  cfblk1/1 -> cfblk4/1, cfblk3/1, cfblk3/2
  cfblk3/1 -> cfblk2/1

== system sampleModel226/cfblk87 ==
  cfblk1 : Inport
  cfblk4 : Inport  Port=2
  cfblk5 : Inport  Port=3
  cfblk3 : Product
  cfblk2 : Outport
  wires:
  cfblk5/1 -> cfblk3/1
  cfblk1/1 -> cfblk2/1
  cfblk4/1 -> cfblk3/2

== system sampleModel226/cfblk88 ==
  cfblk1 : Inport
  cfblk3 : MinMax  Function=max  Inputs=3
  cfblk2 : Outport
  wires:
  cfblk1/1 -> cfblk3/1, cfblk3/2, cfblk3/3
  cfblk3/1 -> cfblk2/1

== system sampleModel226/cfblk89 ==
  cfblk1 : Inport
  cfblk3 : simulink/Discrete/Difference  ICPrevInput=0.0  OutMin=[]  OutMax=[]  OutDataTypeStr=Inherit: Inherit via back propagation  OutDataType=fixdt(1, 16)  OutScaling=2^-10  DoSatur=off
  cfblk4 : MinMax  Function=max
  cfblk5 : Delay  SampleTime=1
  cfblk2 : Outport
  wires:
  cfblk1/1 -> cfblk2/1
  cfblk3/1 -> cfblk4/1
  cfblk4/1 -> cfblk5/1
  cfblk5/1 -> cfblk3/1

== system sampleModel226/cfblk90 ==
  cfblk1 : Inport
  cfblk3 : DiscreteFir  SampleTime=1
  cfblk2 : Outport
  wires:
  cfblk3/1 -> cfblk2/1
  cfblk1/1 -> cfblk3/1

== system sampleModel226/cfblk91 ==
  cfblk1 : Inport
  cfblk3 : slpidlib/PID Controller  Controller=PID  Form=Parallel  TimeDomain=Discrete-time  UseExternalTs=off  SampleTime=1  IntegratorMethod=Forward Euler  FilterMethod=Forward Euler  ControllerParametersSource=internal  P=1  I=1  D=0  UseFilter=on  N=100  TunerSelectOption=Transfer Function Based (PID Tuner App)  InitialConditionSource=internal  InitialConditionForIntegrator=0  InitialConditionForFilter=0  DifferentiatorICPrevScaledInput=0  ExternalReset=none  TrackingMode=off  Kt=1  LimitOutput=off  SatLimitsSource=internal  UpperSaturationLimit=inf  LowerSaturationLimit=-inf  LinearizeAsGain=off  AntiWindupMode=none  Kb=1  POutMin=[]  POutMax=[]  IOutMin=[]  IOutMax=[]  DOutMin=[]  DOutMax=[]  NOutMin=[]  NOutMax=[]  SumOutMin=[]  SumOutMax=[]  SaturationOutMin=[]  SaturationOutMax=[]  PParamMin=[]  PParamMax=[]  IParamMin=[]  IParamMax=[]  DParamMin=[]  DParamMax=[]  NParamMin=[]  NParamMax=[]  KbParamMin=[]  KbParamMax=[]  KtParamMin=[]  KtParamMax=[]  KbOutMin=[]  KbOutMax=[]  KtOutMin=[]  KtOutMax=[]  IntegratorOutMin=[]  IntegratorOutMax=[]  FilterOutMin=[]  FilterOutMax=[]  SumI1OutMin=[]  SumI1OutMax=[]  SumI2OutMin=[]  SumI2OutMax=[]  SumI3OutMin=[]  SumI3OutMax=[]  SumI4OutMin=[]  SumI4OutMax=[]  SumDOutMin=[]  SumDOutMax=[]  DifferentiatorOutMin=[]  DifferentiatorOutMax=[]  FilterDiffOutCoefMin=[]  FilterDiffOutCoefMax=[]  ReciprocalOutMin=[]  ReciprocalOutMax=[]  SumDenOutMin=[]  SumDenOutMax=[]  SumNumOutMin=[]  SumNumOutMax=[]  DivideOutMin=[]  DivideOutMax=[]  UdiffTsProdOutMin=[]  UdiffTsProdOutMax=[]  NTsProdOutMin=[]  NTsProdOutMax=[]  UintegralTsProdOutMin=[]  UintegralTsProdOutMax=[]  UngainTsProdOutMin=[]  UngainTsProdOutMax=[]  IntegratorContinuousStateAttributes=''  IntegratorStateMustResolveToSignalObject=off  IntegratorRTWStateStorageClass=Auto  FilterContinuousStateAttributes=''  FilterStateMustResolveToSignalObject=off  FilterRTWStateStorageClass=Auto  ParallelPVariant=InternalParameters  IdealPVariant=Disabled  IVariant=InternalParameters  DVariant=InternalParameters  IntegratorVariant=Discrete  SatVariant=Disabled  AWVariant=Passthrough  PCopyVariant=Disabled  TRVariant=Disabled  FdbkBlocksVariant=Forward  IdealPFdbkVariant=Disabled  SatFdbkVariant=Disabled  DerivativeFilterVariant=ForwardEulerFilter  NVariant=InternalParameters  NCopyVariant=Disabled  FilterICVariant=InternalICsFilter  IntegratorICVariant=InternalICs  ExternalResetVariant=Disabled  TRSumVariant=Passthrough  SumFdbkVariant=Disabled  SumVariant=Sum_PID  TsampFilterVariant=InternalTs  TsampNgainVariant=Passthrough  TsampIntegralVariant=Passthrough  ExternalSaturationOutDataTypeStr=Inherit: Same as second input
  cfblk4 : Rounding
  cfblk5 : Constant  Value=[-477470430.677754]  SampleTime=1
  cfblk2 : Outport
  wires:
  cfblk5/1 -> cfblk3/1
  cfblk1/1 -> cfblk2/1
  cfblk3/1 -> cfblk4/1

== system sampleModel226/cfblk92 ==
  cfblk1 : Inport
  cfblk3 : Inport  Port=2
  cfblk4 : Inport  Port=3
  cfblk2 : Outport
  wires:
  cfblk1/1 -> cfblk2/1

== system sampleModel226/cfblk93 ==
  cfblk1 : Inport
  cfblk5 : Inport  Port=2
  cfblk3 : Assignment  DiagnosticForDimensions=Warning  IndexOptions=Index vector (dialog)  Indices=1  OutputSizes=1
  cfblk4 : Constant  Value=[48621712.495757]  SampleTime=1
  cfblk2 : Outport
  wires:
  cfblk5/1 -> cfblk2/1
  cfblk1/1 -> cfblk3/1
  cfblk4/1 -> cfblk3/2

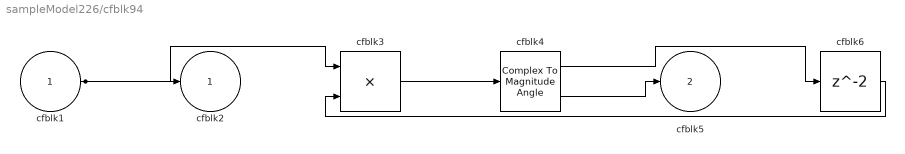
== system sampleModel226/cfblk94 ==
  cfblk1 : Inport
  cfblk3 : Product  Inputs=**
  cfblk4 : ComplexToMagnitudeAngle
  cfblk6 : Delay  SampleTime=1
  cfblk2 : Outport
  cfblk5 : Outport  Port=2
  wires:
  cfblk1/1 -> cfblk3/1, cfblk2/1
  cfblk3/1 -> cfblk4/1
  cfblk4/2 -> cfblk5/1
  cfblk4/1 -> cfblk6/1
  cfblk6/1 -> cfblk3/2
